simulink model "simulacionnolineal2"  (R2017b)
settings: Solver=VariableStepAuto  StartTime=0.0  StopTime=10.0  RelTol=1e-3
settings Model: Creator=alfre  LastModifiedBy=alfre

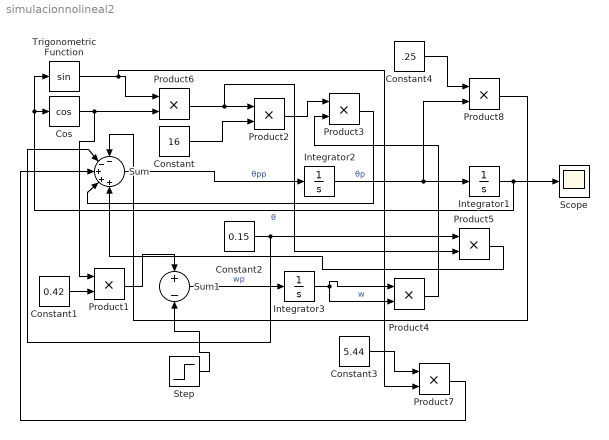
== system simulacionnolineal2 ==
  Constant : Constant  Value=16
  Constant1 : Constant  Value=0.42
  Constant2 : Constant  Value=0.15
  Constant3 : Constant  Value=5.44
  Constant4 : Constant  Value=.25
  Cos : Trigonometry  Operator=cos
  Integrator1 : Integrator
  Integrator2 : Integrator
  Integrator3 : Integrator
  Product{1..8} (8 alike) : Product
  Scope : Scope
  Step : Step  Time=.20  SampleTime=0
  Sum : Sum  Inputs=--+++
  Sum1 : Sum  Inputs=+-
  Trigonometric Function : Trigonometry
  wires:
  Sum/1 -> Integrator2/1  "θpp"
  Constant/1 -> Product2/2
  Cos/1 -> Product1/1, Product6/2
  Integrator2/1 -> Product8/2, Integrator1/1  "θp"
  Integrator1/1 -> Cos/1, Trigonometric Function/1, Scope/1  "θ"
  Step/1 -> Sum1/2
  Constant1/1 -> Product1/2
  Product1/1 -> Sum1/1
  Sum1/1 -> Integrator3/1  "wp"
  Integrator3/1 -> Product4/1, Product4/2  "w"
  Product6/1 -> Product5/2, Product2/1
  Product2/1 -> Product3/1
  Product4/1 -> Product3/2
  Product3/1 -> Sum/4
  Constant2/1 -> Sum/2, Product5/1
  Product5/1 -> Sum/5
  Constant3/1 -> Product7/1
  Product7/1 -> Sum/3
  Constant4/1 -> Product8/1
  Product8/1 -> Sum/1
  Trigonometric Function/1 -> Product7/2, Product6/1
